simulink model "SVPWM_Base_MATLABfcn"  (R2020b)
settings: Solver=ode23tb  StartTime=0.0  StopTime=0.05  MaxStep=0.00001  RelTol=1e-3
libraries: simulink x1
settings Model: Creator=15070  LastModifiedBy=15070

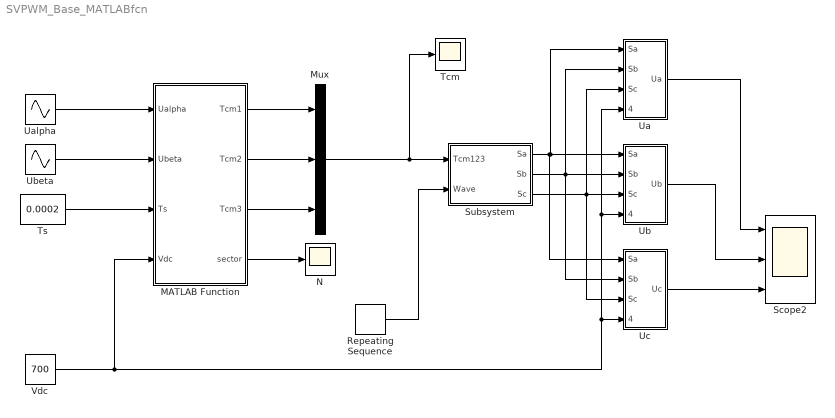
== system SVPWM_Base_MATLABfcn ==
  MATLAB Function : MATLAB Function  TreatAsAtomicUnit=on
  Mux : Mux  Inputs=3
  N : Scope
  Repeating Sequence : simulink/Sources/Repeating Sequence  rep_seq_t=[0 1/10000 1/5000]  rep_seq_y=[0 1/10000 0]
  Scope2 : Scope  NumInputPorts=3
  Subsystem : Subsystem
  Tcm : Scope
  Ts : Constant  Value=0.0002
  Ua : Subsystem
  Ualpha : Sin  Amplitude=200  Frequency=2*50*pi  Phase=pi/2  SampleTime=10e-6
  Ub : Subsystem
  Ubeta : Sin  Amplitude=200  Frequency=2*50*pi  SampleTime=10e-6
  Uc : Subsystem
  Vdc : Constant  Value=700
  wires:
  Vdc/1 -> MATLAB Function/4(Vdc), Ua/4(Vdc), Ub/4(Vdc), Uc/4(Vdc)
  Mux/1 -> Tcm/1, Subsystem/1(Tcm123)
  Repeating Sequence/1 -> Subsystem/2(Wave)
  Subsystem/2(Sb) -> Uc/2(Sb), Ua/2(Sb), Ub/2(Sb)
  Subsystem/1(Sa) -> Uc/1(Sa), Ua/1(Sa), Ub/1(Sa)
  Subsystem/3(Sc) -> Uc/3(Sc), Ua/3(Sc), Ub/3(Sc)
  Ua/1(Ua) -> Scope2/1
  Ub/1(Ub) -> Scope2/2
  Uc/1(Uc) -> Scope2/3
  Ubeta/1 -> MATLAB Function/2(Ubeta)
  Ualpha/1 -> MATLAB Function/1(Ualpha)
  Ts/1 -> MATLAB Function/3(Ts)
  MATLAB Function/4(sector) -> N/1
  MATLAB Function/3(Tcm3) -> Mux/3
  MATLAB Function/2(Tcm2) -> Mux/2
  MATLAB Function/1(Tcm1) -> Mux/1

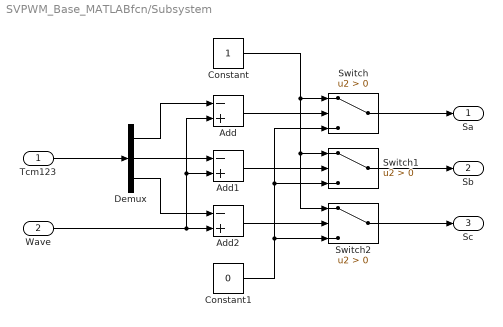
== system SVPWM_Base_MATLABfcn/Subsystem ==
  Tcm123 : Inport
  Wave : Inport  Port=2
  Add : Sum  Inputs=-+
  Add1 : Sum  Inputs=-+
  Add2 : Sum  Inputs=-+
  Constant : Constant
  Constant1 : Constant  Value=0
  Demux : Demux  Outputs=3
  Switch : Switch  Criteria=u2 > Threshold
  Switch1 : Switch  Criteria=u2 > Threshold
  Switch2 : Switch  Criteria=u2 > Threshold
  Sa : Outport
  Sb : Outport  Port=2
  Sc : Outport  Port=3
  wires:
  Constant1/1 -> Switch2/3, Switch/3, Switch1/3
  Wave/1 -> Add1/2, Add/2, Add2/2
  Constant/1 -> Switch1/1, Switch2/1, Switch/1
  Add2/1 -> Switch2/2
  Add1/1 -> Switch1/2
  Tcm123/1 -> Demux/1
  Switch2/1 -> Sc/1
  Switch/1 -> Sa/1
  Add/1 -> Switch/2
  Switch1/1 -> Sb/1
  Demux/2 -> Add1/1
  Demux/3 -> Add2/1
  Demux/1 -> Add/1

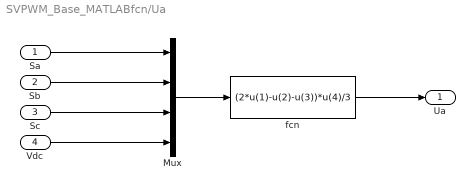
== system SVPWM_Base_MATLABfcn/Ua ==
  Sa : Inport
  Sb : Inport  Port=2
  Sc : Inport  Port=3
  Vdc : Inport  Port=4
  Mux : Mux
  fcn : Fcn  Expr=(2*u(1)-u(2)-u(3))*u(4)/3
  Ua : Outport
  wires:
  Sb/1 -> Mux/2
  Mux/1 -> fcn/1
  Vdc/1 -> Mux/4
  Sc/1 -> Mux/3
  Sa/1 -> Mux/1
  fcn/1 -> Ua/1

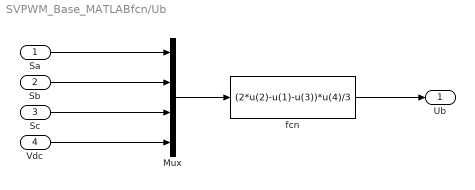
== system SVPWM_Base_MATLABfcn/Ub ==
  Sa : Inport
  Sb : Inport  Port=2
  Sc : Inport  Port=3
  Vdc : Inport  Port=4
  Mux : Mux
  fcn : Fcn  Expr=(2*u(2)-u(1)-u(3))*u(4)/3
  Ub : Outport
  wires:
  Sb/1 -> Mux/2
  Mux/1 -> fcn/1
  Vdc/1 -> Mux/4
  Sc/1 -> Mux/3
  Sa/1 -> Mux/1
  fcn/1 -> Ub/1

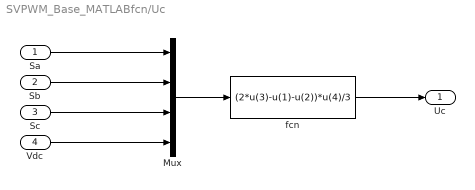
== system SVPWM_Base_MATLABfcn/Uc ==
  Sa : Inport
  Sb : Inport  Port=2
  Sc : Inport  Port=3
  Vdc : Inport  Port=4
  Mux : Mux
  fcn : Fcn  Expr=(2*u(3)-u(1)-u(2))*u(4)/3
  Uc : Outport
  wires:
  Sb/1 -> Mux/2
  Mux/1 -> fcn/1
  Vdc/1 -> Mux/4
  Sc/1 -> Mux/3
  Sa/1 -> Mux/1
  fcn/1 -> Uc/1

== matlab function SVPWM_Base_MATLABfcn/MATLAB Function ==
  data: Ualpha input; Tcm1 output; Ubeta input; Ts input; Vdc input; Tcm2 output; Tcm3 output; sector output
function [Tcm1,Tcm2,Tcm3,sector] = fcn(Ualpha,Ubeta,Ts,Vdc)

sector = 0;
Tcm1 = 0;
Tcm2 = 0;
Tcm3 = 0;

Uref1 = Ubeta;
Uref2 = (sqrt(3) * Ualpha - Ubeta)/2;
Uref3 = (-sqrt(3) * Ualpha - Ubeta)/2;

%===========Sector calculation==========%
if (Uref1>0)
    sector = 1;
end
if (Uref2>0)
    sector = sector + 2;
end
if (Uref3>0)
    sector = sector +4;
end

%==========X Y Z calculation==========%
X = sqrt(3) * Ubeta * Ts / Vdc;
Y = Ts / Vdc * (3/2 * Ualpha + sqrt(3)/2 * Ubeta);
Z = Ts / Vdc * (-3/2 * Ualpha + sqrt(3)/2 * Ubeta);

%==========Duty ration calculation==========%
switch (sector)
    case 1
        T1 = Z;
        T2 = Y;
    case 2
        T1 = Y;
        T2 = -X;
    case 3
        T1 = -Z;
        T2 = X;
    case 4
        T1 = -X;
        T2 = Z;
    case 5
        T1 = X;
        T2 = -Y;
    otherwise
        T1 = -Y;
        T2 = -Z;
end

%==========modulate==========%
if T1 + T2 > Ts
    T1 = T1 / (T1 + T2);
    T2 = T2 / (T1 + T2);
else
    T1 = T1;
    T2 = T2;
end
ta = (Ts - (T1+T2)) /  4.0;
tb = ta + T1/2;
tc = tb + T2/2;

%==========Duty ratio calculation==========%
switch (sector)
    case 1
        Tcm1 = tb;
        Tcm2 = ta;
        Tcm3 = tc;
    case 2
        Tcm1 = ta;
        Tcm2 = tc;
        Tcm3 = tb;
    case 3
        Tcm1 = ta;
        Tcm2 = tb;
        Tcm3 = tc;
    case 4
        Tcm1 = tc;
        Tcm2 = tb;
        Tcm3 = ta;
    case 5
        Tcm1 = tc;
        Tcm2 = ta;
        Tcm3 = tb;
    case 6
        Tcm1 = tb;
        Tcm2 = tc;
        Tcm3 = ta;
end
end
